simulink model "REALTIME_PART3_direct_digital_nominal"  (R2020b)
settings: Solver=ode3  StartTime=0.0  StopTime=5  FixedStep=0.001  RelTol=1e-3
undefined symbols (not defined in the file or in its folder): degs2rpm, denHws, GAMMA0, H0, J0, N_u, N_x, National_Instruments, numHws, PCI, PHI0, sens, step_size, T
libraries: sldrtlib x2
settings Model: ExtModeTrigDuration=6000  Creator=utente  LastModifiedBy=pavarinlau
settings DataIOCC: ReturnWorkspaceOutputs=off
settings RTWCC: Description=Simulink Desktop Real-Time  SystemTargetFile=sldrt.tlc  TemplateMakefile=sldrt.tmf  RTWCompilerOptimization=on
settings CodeAppCC: MaxIdLength=95
settings SimulinkDesktopRealTimeCC: TargetPreCompLibLocation=C:\Program Files\MATLAB\R2020b\toolbox\sldrt\lib\win64

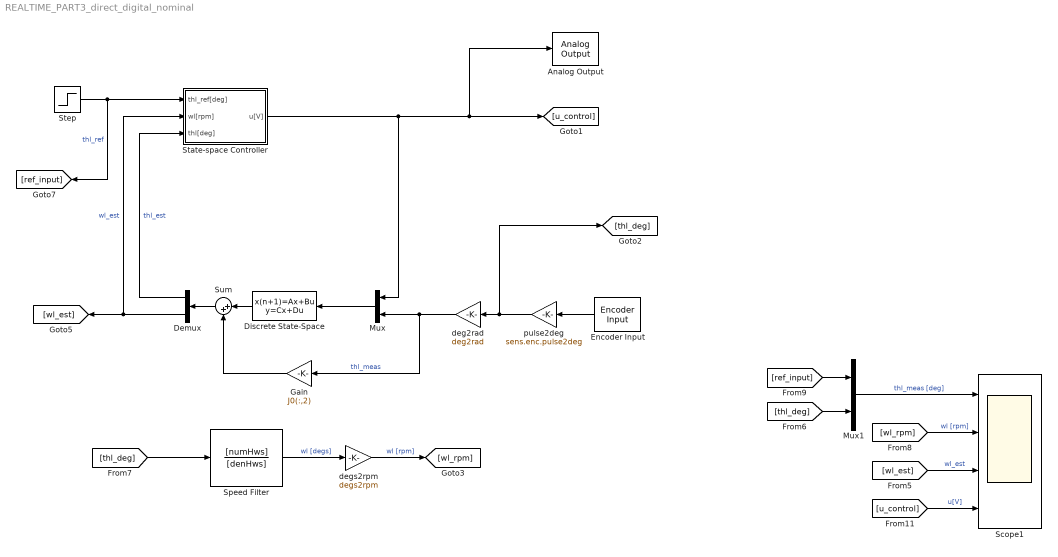
== system REALTIME_PART3_direct_digital_nominal ==
  Analog Output : sldrtlib/Analog Output  SampleTime=-1  MaxMissedTicks=10  ShowMissedTicks=off  YieldWhenWaiting=off  DrvName=National_Instruments/PCI-6221  DrvAddress=4294967295  DrvOptions=[0 0 0 2 0]  Channels=1  RangeMode=1  VoltRange=1  InitialValue=0  FinalValue=0
      settings: AttributesFormatString=National Instruments\nPCI-6221 [auto]
  Demux : Demux  Outputs=2
  Discrete State-Space : DiscreteStateSpace  A=PHI0  B=GAMMA0  C=H0  D=[0 0;0 0]  SampleTime=T
  Encoder Input : sldrtlib/Encoder Input  SampleTime=T  MaxMissedTicks=10  ShowMissedTicks=off  YieldWhenWaiting=off  DrvName=National_Instruments/PCI-6221  DrvAddress=4294967295  DrvOptions=[0 0 0 2 0]  Channels=1  QuadMode=3  IndexPulse=1  InputFilter=Inf  DataType=1
      settings: AttributesFormatString=National Instruments\nPCI-6221 [auto]
  Gain : Gain  Gain=J0(:,2)
  Mux : Mux  Inputs=2
  Mux1 : Mux  Inputs=2
  Scope1 : Scope  NumInputPorts=4
  Speed Filter : TransferFcn  Numerator=[numHws]  Denominator=[denHws]
  State-space Controller : Subsystem
  Step : Step  After=step_size  SampleTime=T
  Sum : Sum  Inputs=|++
  deg2rad : Gain  Gain=deg2rad
  degs2rpm : Gain  Gain=degs2rpm
  pulse2deg : Gain  Gain=sens.enc.pulse2deg
  wires:
  Encoder Input/1 -> pulse2deg/1
  Step/1 -> [ref_input], State-space Controller/1(thl_ref[deg])  "thl_ref"
  pulse2deg/1 -> [thl_deg], deg2rad/1
  deg2rad/1 -> Gain/1, Mux/2  "thl_meas"
  Demux/1 -> State-space Controller/3(thl[deg])  "thl_est"
  Demux/2 -> State-space Controller/2(wl[rpm]), [wl_est]  "wl_est"
  Mux/1 -> Discrete State-Space/1
  State-space Controller/1(u[V]) -> Analog Output/1, [u_control], Mux/1
  [thl_deg] -> Speed Filter/1
  degs2rpm/1 -> [wl_rpm]  "wl [rpm]"
  Speed Filter/1 -> degs2rpm/1  "wl [degs]"
  [u_control] -> Scope1/4  "u[V]"
  Mux1/1 -> Scope1/1  "thl_meas [deg]"
  [wl_rpm] -> Scope1/2  "wl [rpm]"
  [ref_input] -> Mux1/1
  [wl_est] -> Scope1/3  "wl_est"
  [thl_deg] -> Mux1/2
  Discrete State-Space/1 -> Sum/1
  Sum/1 -> Demux/1
  Gain/1 -> Sum/2

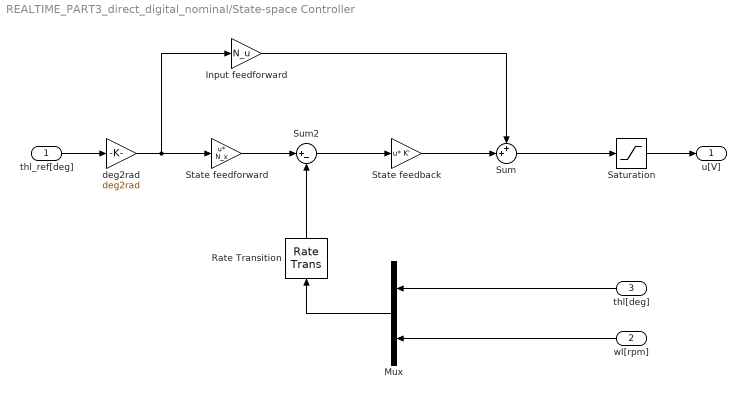
== system REALTIME_PART3_direct_digital_nominal/State-space Controller ==
  thl_ref[deg] : Inport
  wl[rpm] : Inport  Port=2
  thl[deg] : Inport  Port=3
  Input feedforward : Gain  Gain=N_u
  Mux : Mux  Inputs=2
  Rate Transition : RateTransition
  Saturation : Saturate  UpperLimit=10  LowerLimit=-10
  State feedback : Gain  Gain=K'  Multiplication=Matrix(u*K)
  "State feedforward\t" : Gain  Gain=N_x  Multiplication=Matrix(u*K)
  Sum : Sum  Inputs=++|
  Sum2 : Sum  Inputs=|+-
  deg2rad : Gain  Gain=deg2rad
  u[V] : Outport
  wires:
  thl_ref[deg]/1 -> deg2rad/1
  deg2rad/1 -> Input feedforward/1, "State feedforward\t"/1
  State feedback/1 -> Sum/2
  "State feedforward\t"/1 -> Sum2/1
  Sum2/1 -> State feedback/1
  Input feedforward/1 -> Sum/1
  Sum/1 -> Saturation/1
  Saturation/1 -> u[V]/1
  thl[deg]/1 -> Mux/1
  wl[rpm]/1 -> Mux/2
  Mux/1 -> Rate Transition/1
  Rate Transition/1 -> Sum2/2
